simulink model "Tipo4_v4"  (R2018b)
settings: Solver=FixedStepDiscrete  StartTime=0.0  StopTime=50.3  MaxStep=50e-6  RelTol=1e-3
PreLoadFcn:
  | Ts=2e-6;
InitFcn:
  | %xInitial = init_power_wind_dfig_det;
  | Ts=2e-6;
undefined symbols (not defined in the file): D1, Delta, DiscIntNeverNeededParam, find_system
libraries: powerlib x144, simulink x110, powerlib_meascontrol x83, simulink_extras x6, powerlib_extras x4
(part 3 of 6)

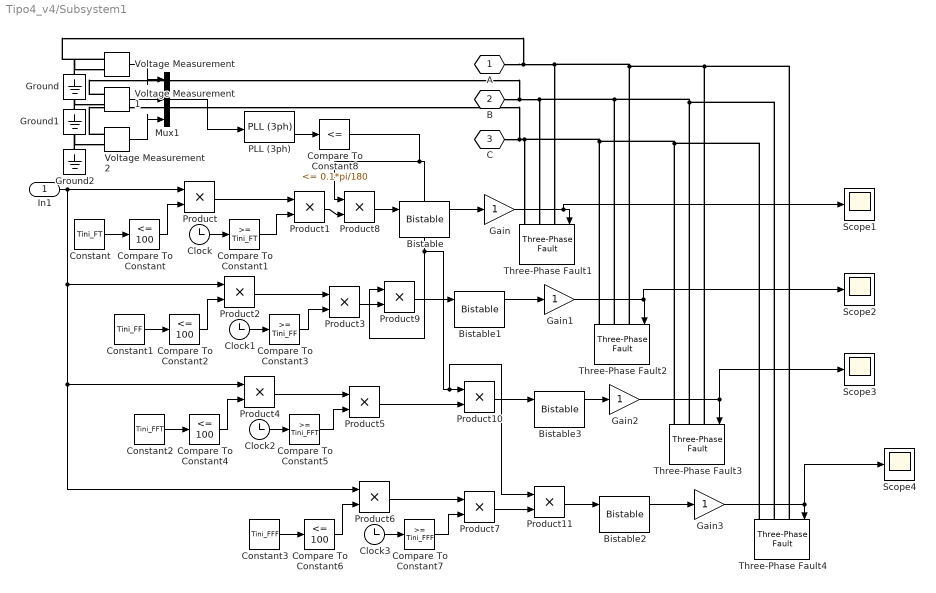
== system Tipo4_v4/Subsystem1 ==
  In1 : Inport
  Bistable{,1..3} (4 alike) : powerlib_meascontrol/Logic/Bistable  Qpriority=Set  ic=0  Ts=Ts
      settings: SourceProductName=Simscape Power Systems  SourceProductBaseCode=PS
  Clock{,1..3} (4 alike) : Clock
  Compare To Constant{,2,4,6} (4 alike) : simulink/Logic and Bit Operations/Compare To Constant  relop=<=  const=100  OutDataTypeStr=uint8
  Compare To Constant1 : simulink/Logic and Bit Operations/Compare To Constant  relop=>=  const=Tini_FT  OutDataTypeStr=uint8
  Compare To Constant3 : simulink/Logic and Bit Operations/Compare To Constant  relop=>=  const=Tini_FF  OutDataTypeStr=uint8
  Compare To Constant5 : simulink/Logic and Bit Operations/Compare To Constant  relop=>=  const=Tini_FFT  OutDataTypeStr=uint8
  Compare To Constant7 : simulink/Logic and Bit Operations/Compare To Constant  relop=>=  const=Tini_FFF  OutDataTypeStr=uint8
  Compare To Constant8 : simulink/Logic and Bit Operations/Compare To Constant  relop=<=  const=0.1*pi/180  OutDataTypeStr=uint8
  Constant : Constant  Value=Tini_FT
  Constant1 : Constant  Value=Tini_FF
  Constant2 : Constant  Value=Tini_FFT
  Constant3 : Constant  Value=Tini_FFF
  Gain{,1..3} (4 alike) : Gain  OutDataTypeStr=double
  Ground : powerlib/Elements/Ground  LConnTagsString=a
  Ground1 : powerlib/Elements/Ground  LConnTagsString=a
  Ground2 : powerlib/Elements/Ground  LConnTagsString=a
  Mux1 : Mux  Inputs=3
  PLL (3ph) : powerlib_meascontrol/PLL/PLL (3ph)  Fmin=60  Par_Init=[0, 60]  ParK=[180, 3200, 1]  TcD=1e-4  MaxRateChangeFreq=12  FilterCutOffFreq=25  Ts=Ts  AGC=on
  Product{,2..7} (7 alike) : Product
  Product{1,8..11} (5 alike) : Product  RndMeth=Ceiling
  Scope{1..4} (4 alike) : Scope
  Three-Phase Fault1 : powerlib/Elements/Three-Phase Fault  InitialStates=0  FaultA=on  FaultB=off  FaultC=off  GroundFault=on  SwitchTimes=[900 1000]  External=on  SwitchStatus=NaN  FaultResistance=R_falta  GroundResistance=R_falta  SnubberResistance=1e6  SnubberCapacitance=inf  Measurements=None
  Three-Phase Fault2 : powerlib/Elements/Three-Phase Fault  InitialStates=0  FaultA=on  FaultB=on  FaultC=off  GroundFault=off  SwitchTimes=[900 1000]  External=on  SwitchStatus=NaN  FaultResistance=R_falta  GroundResistance=1e-12  SnubberResistance=1e6  SnubberCapacitance=inf  Measurements=None
  Three-Phase Fault3 : powerlib/Elements/Three-Phase Fault  InitialStates=0  FaultA=on  FaultB=on  FaultC=off  GroundFault=on  SwitchTimes=[900 1000]  External=on  SwitchStatus=NaN  FaultResistance=R_falta  GroundResistance=R_falta  SnubberResistance=1e6  SnubberCapacitance=inf  Measurements=None
  Three-Phase Fault4 : powerlib/Elements/Three-Phase Fault  InitialStates=0  FaultA=on  FaultB=on  FaultC=on  GroundFault=on  SwitchTimes=[900 1000]  External=on  SwitchStatus=NaN  FaultResistance=R_falta  GroundResistance=R_falta  SnubberResistance=1e6  SnubberCapacitance=inf  Measurements=None
  Voltage Measurement : powerlib/Measurements/Voltage Measurement  PhasorSimulation=off  OutputType=Complex  PSBequivalent=0
  Voltage Measurement1 : powerlib/Measurements/Voltage Measurement  PhasorSimulation=off  OutputType=Complex  PSBequivalent=0
  Voltage Measurement2 : powerlib/Measurements/Voltage Measurement  PhasorSimulation=off  OutputType=Complex  PSBequivalent=0
  A : PMIOPort  Tag=PMCPort  Side=Right
  B : PMIOPort  Tag=PMCPort  Port=2  Side=Right
  C : PMIOPort  Tag=PMCPort  Port=3  Side=Right
  wires:
  Clock/1 -> Compare To Constant1/1
  Product2/1 -> Product3/1
  Constant1/1 -> Compare To Constant2/1
  Product/1 -> Product1/1
  Compare To Constant2/1 -> Product2/2
  Constant2/1 -> Compare To Constant4/1
  Clock2/1 -> Compare To Constant5/1
  Compare To Constant4/1 -> Product4/2
  Clock1/1 -> Compare To Constant3/1
  Compare To Constant5/1 -> Product5/2
  In1/1 -> Product/1, Product2/1, Product4/1, Product6/1
  Clock3/1 -> Compare To Constant7/1
  Constant3/1 -> Compare To Constant6/1
  Compare To Constant6/1 -> Product6/2
  Product6/1 -> Product7/1
  Compare To Constant7/1 -> Product7/2
  Compare To Constant3/1 -> Product3/2
  Constant/1 -> Compare To Constant/1
  Compare To Constant/1 -> Product/2
  Compare To Constant1/1 -> Product1/2
  Product4/1 -> Product5/1
  Product1/1 -> Product8/2
  Product8/1 -> Bistable/1
  Product3/1 -> Product9/2
  Product5/1 -> Product10/2
  Product7/1 -> Product11/2
  Compare To Constant8/1 -> Product11/1, Product10/1, Product9/1, Product8/1
  PLL (3ph)/2 -> Compare To Constant8/1
  Voltage Measurement1/1 -> Mux1/2
  Voltage Measurement/1 -> Mux1/1
  Voltage Measurement2/1 -> Mux1/3
  Mux1/1 -> PLL (3ph)/1
  Gain/1 -> Scope1/1, Three-Phase Fault1/1
  Gain1/1 -> Scope2/1, Three-Phase Fault2/1
  Gain2/1 -> Three-Phase Fault3/1, Scope3/1
  Gain3/1 -> Scope4/1, Three-Phase Fault4/1
  Bistable/1 -> Gain/1
  Product9/1 -> Bistable1/1
  Bistable1/1 -> Gain1/1
  Bistable3/1 -> Gain2/1
  Product10/1 -> Bistable3/1
  Product11/1 -> Bistable2/1
  Bistable2/1 -> Gain3/1
  connections:
  Voltage Measurement1/LConn1 -- B/RConn1 -- Three-Phase Fault1/LConn2 -- Three-Phase Fault2/LConn2 -- Three-Phase Fault3/LConn2 -- Three-Phase Fault4/LConn2
  Voltage Measurement2/LConn1 -- C/RConn1 -- Three-Phase Fault4/LConn3 -- Three-Phase Fault3/LConn3 -- Three-Phase Fault2/LConn3 -- Three-Phase Fault1/LConn3
  A/RConn1 -- Voltage Measurement/LConn1 -- Three-Phase Fault1/LConn1 -- Three-Phase Fault2/LConn1 -- Three-Phase Fault3/LConn1 -- Three-Phase Fault4/LConn1
  Ground/LConn1 -- Voltage Measurement/LConn2
  Ground1/LConn1 -- Voltage Measurement1/LConn2
  Ground2/LConn1 -- Voltage Measurement2/LConn2

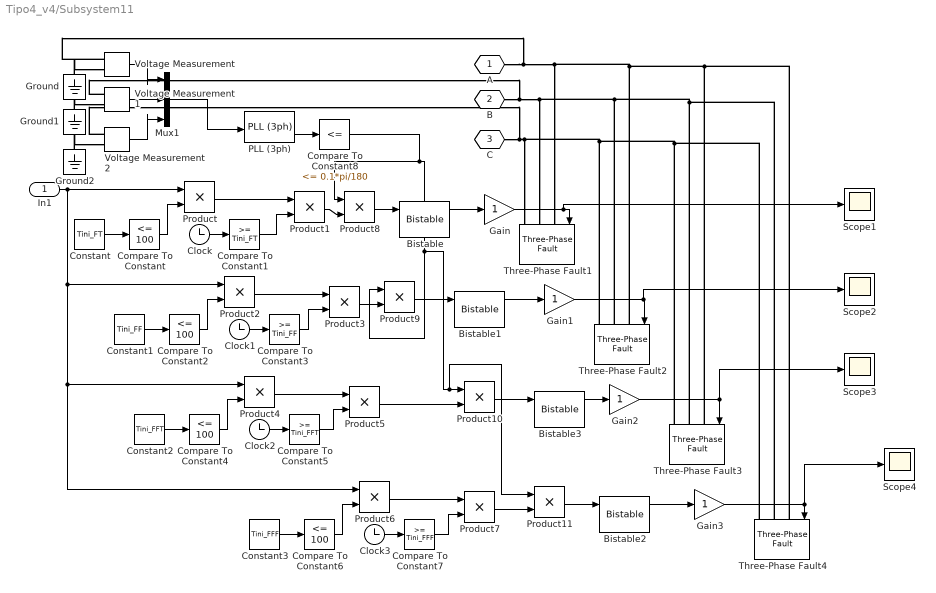
== system Tipo4_v4/Subsystem11 ==
  In1 : Inport
  Bistable{,1..3} (4 alike) : powerlib_meascontrol/Logic/Bistable  Qpriority=Set  ic=0  Ts=Ts
      settings: SourceProductName=Simscape Power Systems  SourceProductBaseCode=PS
  Clock{,1..3} (4 alike) : Clock
  Compare To Constant{,2,4,6} (4 alike) : simulink/Logic and Bit Operations/Compare To Constant  relop=<=  const=100  OutDataTypeStr=uint8
  Compare To Constant1 : simulink/Logic and Bit Operations/Compare To Constant  relop=>=  const=Tini_FT  OutDataTypeStr=uint8
  Compare To Constant3 : simulink/Logic and Bit Operations/Compare To Constant  relop=>=  const=Tini_FF  OutDataTypeStr=uint8
  Compare To Constant5 : simulink/Logic and Bit Operations/Compare To Constant  relop=>=  const=Tini_FFT  OutDataTypeStr=uint8
  Compare To Constant7 : simulink/Logic and Bit Operations/Compare To Constant  relop=>=  const=Tini_FFF  OutDataTypeStr=uint8
  Compare To Constant8 : simulink/Logic and Bit Operations/Compare To Constant  relop=<=  const=0.1*pi/180  OutDataTypeStr=uint8
  Constant : Constant  Value=Tini_FT
  Constant1 : Constant  Value=Tini_FF
  Constant2 : Constant  Value=Tini_FFT
  Constant3 : Constant  Value=Tini_FFF
  Gain{,1..3} (4 alike) : Gain  OutDataTypeStr=double
  Ground : powerlib/Elements/Ground  LConnTagsString=a
  Ground1 : powerlib/Elements/Ground  LConnTagsString=a
  Ground2 : powerlib/Elements/Ground  LConnTagsString=a
  Mux1 : Mux  Inputs=3
  PLL (3ph) : powerlib_meascontrol/PLL/PLL (3ph)  Fmin=60  Par_Init=[0, 60]  ParK=[180, 3200, 1]  TcD=1e-4  MaxRateChangeFreq=12  FilterCutOffFreq=25  Ts=Ts  AGC=on
  Product{,2..7} (7 alike) : Product
  Product{1,8..11} (5 alike) : Product  RndMeth=Ceiling
  Scope{1..4} (4 alike) : Scope
  Three-Phase Fault1 : powerlib/Elements/Three-Phase Fault  InitialStates=0  FaultA=on  FaultB=off  FaultC=off  GroundFault=on  SwitchTimes=[900 1000]  External=on  SwitchStatus=NaN  FaultResistance=R_falta  GroundResistance=R_falta  SnubberResistance=1e6  SnubberCapacitance=inf  Measurements=None
  Three-Phase Fault2 : powerlib/Elements/Three-Phase Fault  InitialStates=0  FaultA=on  FaultB=on  FaultC=off  GroundFault=off  SwitchTimes=[900 1000]  External=on  SwitchStatus=NaN  FaultResistance=R_falta  GroundResistance=1e-12  SnubberResistance=1e6  SnubberCapacitance=inf  Measurements=None
  Three-Phase Fault3 : powerlib/Elements/Three-Phase Fault  InitialStates=0  FaultA=on  FaultB=on  FaultC=off  GroundFault=on  SwitchTimes=[900 1000]  External=on  SwitchStatus=NaN  FaultResistance=R_falta  GroundResistance=R_falta  SnubberResistance=1e6  SnubberCapacitance=inf  Measurements=None
  Three-Phase Fault4 : powerlib/Elements/Three-Phase Fault  InitialStates=0  FaultA=on  FaultB=on  FaultC=on  GroundFault=on  SwitchTimes=[900 1000]  External=on  SwitchStatus=NaN  FaultResistance=R_falta  GroundResistance=R_falta  SnubberResistance=1e6  SnubberCapacitance=inf  Measurements=None
  Voltage Measurement : powerlib/Measurements/Voltage Measurement  PhasorSimulation=off  OutputType=Complex  PSBequivalent=0
  Voltage Measurement1 : powerlib/Measurements/Voltage Measurement  PhasorSimulation=off  OutputType=Complex  PSBequivalent=0
  Voltage Measurement2 : powerlib/Measurements/Voltage Measurement  PhasorSimulation=off  OutputType=Complex  PSBequivalent=0
  A : PMIOPort  Tag=PMCPort  Side=Right
  B : PMIOPort  Tag=PMCPort  Port=2  Side=Right
  C : PMIOPort  Tag=PMCPort  Port=3  Side=Right
  wires:
  Clock/1 -> Compare To Constant1/1
  Product2/1 -> Product3/1
  Constant1/1 -> Compare To Constant2/1
  Product/1 -> Product1/1
  Compare To Constant2/1 -> Product2/2
  Constant2/1 -> Compare To Constant4/1
  Clock2/1 -> Compare To Constant5/1
  Compare To Constant4/1 -> Product4/2
  Clock1/1 -> Compare To Constant3/1
  Compare To Constant5/1 -> Product5/2
  In1/1 -> Product/1, Product2/1, Product4/1, Product6/1
  Clock3/1 -> Compare To Constant7/1
  Constant3/1 -> Compare To Constant6/1
  Compare To Constant6/1 -> Product6/2
  Product6/1 -> Product7/1
  Compare To Constant7/1 -> Product7/2
  Compare To Constant3/1 -> Product3/2
  Constant/1 -> Compare To Constant/1
  Compare To Constant/1 -> Product/2
  Compare To Constant1/1 -> Product1/2
  Product4/1 -> Product5/1
  Product1/1 -> Product8/2
  Product8/1 -> Bistable/1
  Product3/1 -> Product9/2
  Product5/1 -> Product10/2
  Product7/1 -> Product11/2
  Compare To Constant8/1 -> Product11/1, Product10/1, Product9/1, Product8/1
  PLL (3ph)/2 -> Compare To Constant8/1
  Voltage Measurement1/1 -> Mux1/2
  Voltage Measurement/1 -> Mux1/1
  Voltage Measurement2/1 -> Mux1/3
  Mux1/1 -> PLL (3ph)/1
  Gain/1 -> Scope1/1, Three-Phase Fault1/1
  Gain1/1 -> Scope2/1, Three-Phase Fault2/1
  Gain2/1 -> Three-Phase Fault3/1, Scope3/1
  Gain3/1 -> Scope4/1, Three-Phase Fault4/1
  Bistable/1 -> Gain/1
  Product9/1 -> Bistable1/1
  Bistable1/1 -> Gain1/1
  Bistable3/1 -> Gain2/1
  Product10/1 -> Bistable3/1
  Product11/1 -> Bistable2/1
  Bistable2/1 -> Gain3/1
  connections:
  Voltage Measurement1/LConn1 -- B/RConn1 -- Three-Phase Fault1/LConn2 -- Three-Phase Fault2/LConn2 -- Three-Phase Fault3/LConn2 -- Three-Phase Fault4/LConn2
  Voltage Measurement2/LConn1 -- C/RConn1 -- Three-Phase Fault4/LConn3 -- Three-Phase Fault3/LConn3 -- Three-Phase Fault2/LConn3 -- Three-Phase Fault1/LConn3
  A/RConn1 -- Voltage Measurement/LConn1 -- Three-Phase Fault1/LConn1 -- Three-Phase Fault2/LConn1 -- Three-Phase Fault3/LConn1 -- Three-Phase Fault4/LConn1
  Ground/LConn1 -- Voltage Measurement/LConn2
  Ground1/LConn1 -- Voltage Measurement1/LConn2
  Ground2/LConn1 -- Voltage Measurement2/LConn2

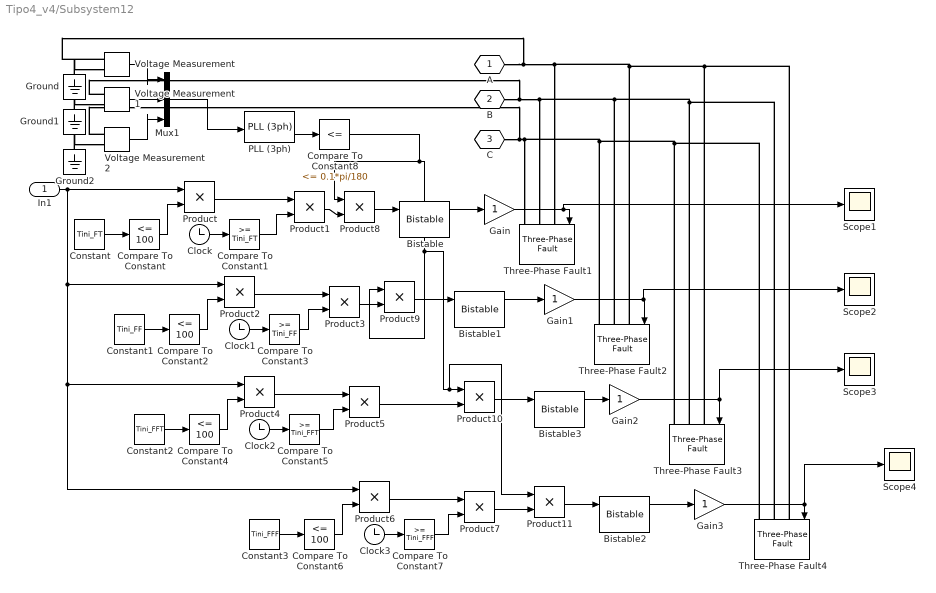
== system Tipo4_v4/Subsystem12 ==
  In1 : Inport
  Bistable{,1..3} (4 alike) : powerlib_meascontrol/Logic/Bistable  Qpriority=Set  ic=0  Ts=Ts
      settings: SourceProductName=Simscape Power Systems  SourceProductBaseCode=PS
  Clock{,1..3} (4 alike) : Clock
  Compare To Constant{,2,4,6} (4 alike) : simulink/Logic and Bit Operations/Compare To Constant  relop=<=  const=100  OutDataTypeStr=uint8
  Compare To Constant1 : simulink/Logic and Bit Operations/Compare To Constant  relop=>=  const=Tini_FT  OutDataTypeStr=uint8
  Compare To Constant3 : simulink/Logic and Bit Operations/Compare To Constant  relop=>=  const=Tini_FF  OutDataTypeStr=uint8
  Compare To Constant5 : simulink/Logic and Bit Operations/Compare To Constant  relop=>=  const=Tini_FFT  OutDataTypeStr=uint8
  Compare To Constant7 : simulink/Logic and Bit Operations/Compare To Constant  relop=>=  const=Tini_FFF  OutDataTypeStr=uint8
  Compare To Constant8 : simulink/Logic and Bit Operations/Compare To Constant  relop=<=  const=0.1*pi/180  OutDataTypeStr=uint8
  Constant : Constant  Value=Tini_FT
  Constant1 : Constant  Value=Tini_FF
  Constant2 : Constant  Value=Tini_FFT
  Constant3 : Constant  Value=Tini_FFF
  Gain{,1..3} (4 alike) : Gain  OutDataTypeStr=double
  Ground : powerlib/Elements/Ground  LConnTagsString=a
  Ground1 : powerlib/Elements/Ground  LConnTagsString=a
  Ground2 : powerlib/Elements/Ground  LConnTagsString=a
  Mux1 : Mux  Inputs=3
  PLL (3ph) : powerlib_meascontrol/PLL/PLL (3ph)  Fmin=60  Par_Init=[0, 60]  ParK=[180, 3200, 1]  TcD=1e-4  MaxRateChangeFreq=12  FilterCutOffFreq=25  Ts=Ts  AGC=on
  Product{,2..7} (7 alike) : Product
  Product{1,8..11} (5 alike) : Product  RndMeth=Ceiling
  Scope{1..4} (4 alike) : Scope
  Three-Phase Fault1 : powerlib/Elements/Three-Phase Fault  InitialStates=0  FaultA=on  FaultB=off  FaultC=off  GroundFault=on  SwitchTimes=[900 1000]  External=on  SwitchStatus=NaN  FaultResistance=R_falta  GroundResistance=R_falta  SnubberResistance=1e6  SnubberCapacitance=inf  Measurements=None
  Three-Phase Fault2 : powerlib/Elements/Three-Phase Fault  InitialStates=0  FaultA=on  FaultB=on  FaultC=off  GroundFault=off  SwitchTimes=[900 1000]  External=on  SwitchStatus=NaN  FaultResistance=R_falta  GroundResistance=1e-12  SnubberResistance=1e6  SnubberCapacitance=inf  Measurements=None
  Three-Phase Fault3 : powerlib/Elements/Three-Phase Fault  InitialStates=0  FaultA=on  FaultB=on  FaultC=off  GroundFault=on  SwitchTimes=[900 1000]  External=on  SwitchStatus=NaN  FaultResistance=R_falta  GroundResistance=R_falta  SnubberResistance=1e6  SnubberCapacitance=inf  Measurements=None
  Three-Phase Fault4 : powerlib/Elements/Three-Phase Fault  InitialStates=0  FaultA=on  FaultB=on  FaultC=on  GroundFault=on  SwitchTimes=[900 1000]  External=on  SwitchStatus=NaN  FaultResistance=R_falta  GroundResistance=R_falta  SnubberResistance=1e6  SnubberCapacitance=inf  Measurements=None
  Voltage Measurement : powerlib/Measurements/Voltage Measurement  PhasorSimulation=off  OutputType=Complex  PSBequivalent=0
  Voltage Measurement1 : powerlib/Measurements/Voltage Measurement  PhasorSimulation=off  OutputType=Complex  PSBequivalent=0
  Voltage Measurement2 : powerlib/Measurements/Voltage Measurement  PhasorSimulation=off  OutputType=Complex  PSBequivalent=0
  A : PMIOPort  Tag=PMCPort  Side=Right
  B : PMIOPort  Tag=PMCPort  Port=2  Side=Right
  C : PMIOPort  Tag=PMCPort  Port=3  Side=Right
  wires:
  Clock/1 -> Compare To Constant1/1
  Product2/1 -> Product3/1
  Constant1/1 -> Compare To Constant2/1
  Product/1 -> Product1/1
  Compare To Constant2/1 -> Product2/2
  Constant2/1 -> Compare To Constant4/1
  Clock2/1 -> Compare To Constant5/1
  Compare To Constant4/1 -> Product4/2
  Clock1/1 -> Compare To Constant3/1
  Compare To Constant5/1 -> Product5/2
  In1/1 -> Product/1, Product2/1, Product4/1, Product6/1
  Clock3/1 -> Compare To Constant7/1
  Constant3/1 -> Compare To Constant6/1
  Compare To Constant6/1 -> Product6/2
  Product6/1 -> Product7/1
  Compare To Constant7/1 -> Product7/2
  Compare To Constant3/1 -> Product3/2
  Constant/1 -> Compare To Constant/1
  Compare To Constant/1 -> Product/2
  Compare To Constant1/1 -> Product1/2
  Product4/1 -> Product5/1
  Product1/1 -> Product8/2
  Product8/1 -> Bistable/1
  Product3/1 -> Product9/2
  Product5/1 -> Product10/2
  Product7/1 -> Product11/2
  Compare To Constant8/1 -> Product11/1, Product10/1, Product9/1, Product8/1
  PLL (3ph)/2 -> Compare To Constant8/1
  Voltage Measurement1/1 -> Mux1/2
  Voltage Measurement/1 -> Mux1/1
  Voltage Measurement2/1 -> Mux1/3
  Mux1/1 -> PLL (3ph)/1
  Gain/1 -> Scope1/1, Three-Phase Fault1/1
  Gain1/1 -> Scope2/1, Three-Phase Fault2/1
  Gain2/1 -> Three-Phase Fault3/1, Scope3/1
  Gain3/1 -> Scope4/1, Three-Phase Fault4/1
  Bistable/1 -> Gain/1
  Product9/1 -> Bistable1/1
  Bistable1/1 -> Gain1/1
  Bistable3/1 -> Gain2/1
  Product10/1 -> Bistable3/1
  Product11/1 -> Bistable2/1
  Bistable2/1 -> Gain3/1
  connections:
  Voltage Measurement1/LConn1 -- B/RConn1 -- Three-Phase Fault1/LConn2 -- Three-Phase Fault2/LConn2 -- Three-Phase Fault3/LConn2 -- Three-Phase Fault4/LConn2
  Voltage Measurement2/LConn1 -- C/RConn1 -- Three-Phase Fault4/LConn3 -- Three-Phase Fault3/LConn3 -- Three-Phase Fault2/LConn3 -- Three-Phase Fault1/LConn3
  A/RConn1 -- Voltage Measurement/LConn1 -- Three-Phase Fault1/LConn1 -- Three-Phase Fault2/LConn1 -- Three-Phase Fault3/LConn1 -- Three-Phase Fault4/LConn1
  Ground/LConn1 -- Voltage Measurement/LConn2
  Ground1/LConn1 -- Voltage Measurement1/LConn2
  Ground2/LConn1 -- Voltage Measurement2/LConn2

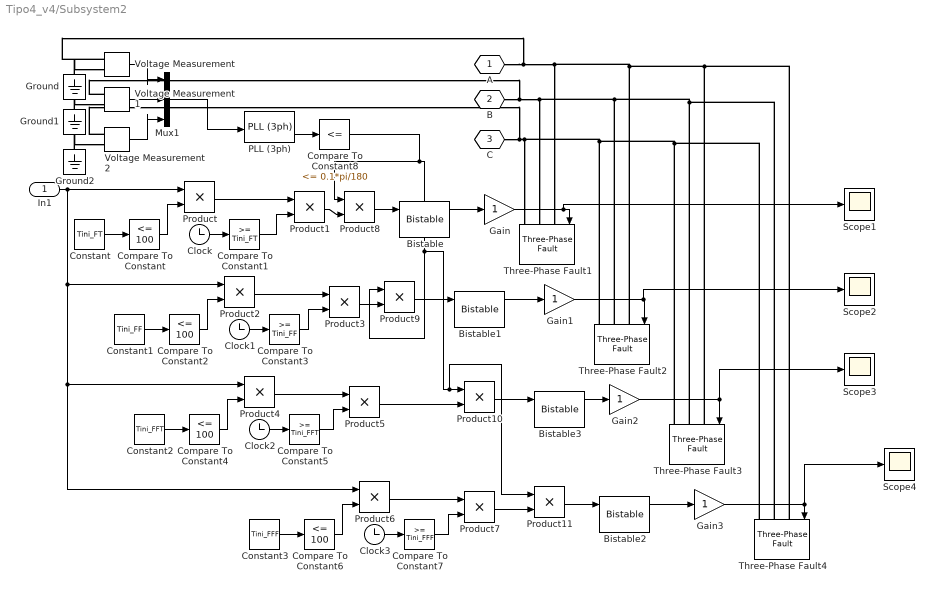
== system Tipo4_v4/Subsystem2 ==
  In1 : Inport
  Bistable{,1..3} (4 alike) : powerlib_meascontrol/Logic/Bistable  Qpriority=Set  ic=0  Ts=Ts
      settings: SourceProductName=Simscape Power Systems  SourceProductBaseCode=PS
  Clock{,1..3} (4 alike) : Clock
  Compare To Constant{,2,4,6} (4 alike) : simulink/Logic and Bit Operations/Compare To Constant  relop=<=  const=100  OutDataTypeStr=uint8
  Compare To Constant1 : simulink/Logic and Bit Operations/Compare To Constant  relop=>=  const=Tini_FT  OutDataTypeStr=uint8
  Compare To Constant3 : simulink/Logic and Bit Operations/Compare To Constant  relop=>=  const=Tini_FF  OutDataTypeStr=uint8
  Compare To Constant5 : simulink/Logic and Bit Operations/Compare To Constant  relop=>=  const=Tini_FFT  OutDataTypeStr=uint8
  Compare To Constant7 : simulink/Logic and Bit Operations/Compare To Constant  relop=>=  const=Tini_FFF  OutDataTypeStr=uint8
  Compare To Constant8 : simulink/Logic and Bit Operations/Compare To Constant  relop=<=  const=0.1*pi/180  OutDataTypeStr=uint8
  Constant : Constant  Value=Tini_FT
  Constant1 : Constant  Value=Tini_FF
  Constant2 : Constant  Value=Tini_FFT
  Constant3 : Constant  Value=Tini_FFF
  Gain{,1..3} (4 alike) : Gain  OutDataTypeStr=double
  Ground : powerlib/Elements/Ground  LConnTagsString=a
  Ground1 : powerlib/Elements/Ground  LConnTagsString=a
  Ground2 : powerlib/Elements/Ground  LConnTagsString=a
  Mux1 : Mux  Inputs=3
  PLL (3ph) : powerlib_meascontrol/PLL/PLL (3ph)  Fmin=60  Par_Init=[0, 60]  ParK=[180, 3200, 1]  TcD=1e-4  MaxRateChangeFreq=12  FilterCutOffFreq=25  Ts=Ts  AGC=on
  Product{,2..7} (7 alike) : Product
  Product{1,8..11} (5 alike) : Product  RndMeth=Ceiling
  Scope{1..4} (4 alike) : Scope
  Three-Phase Fault1 : powerlib/Elements/Three-Phase Fault  InitialStates=0  FaultA=on  FaultB=off  FaultC=off  GroundFault=on  SwitchTimes=[900 1000]  External=on  SwitchStatus=NaN  FaultResistance=R_falta  GroundResistance=R_falta  SnubberResistance=1e6  SnubberCapacitance=inf  Measurements=None
  Three-Phase Fault2 : powerlib/Elements/Three-Phase Fault  InitialStates=0  FaultA=on  FaultB=on  FaultC=off  GroundFault=off  SwitchTimes=[900 1000]  External=on  SwitchStatus=NaN  FaultResistance=R_falta  GroundResistance=1e-12  SnubberResistance=1e6  SnubberCapacitance=inf  Measurements=None
  Three-Phase Fault3 : powerlib/Elements/Three-Phase Fault  InitialStates=0  FaultA=on  FaultB=on  FaultC=off  GroundFault=on  SwitchTimes=[900 1000]  External=on  SwitchStatus=NaN  FaultResistance=R_falta  GroundResistance=R_falta  SnubberResistance=1e6  SnubberCapacitance=inf  Measurements=None
  Three-Phase Fault4 : powerlib/Elements/Three-Phase Fault  InitialStates=0  FaultA=on  FaultB=on  FaultC=on  GroundFault=on  SwitchTimes=[900 1000]  External=on  SwitchStatus=NaN  FaultResistance=R_falta  GroundResistance=R_falta  SnubberResistance=1e6  SnubberCapacitance=inf  Measurements=None
  Voltage Measurement : powerlib/Measurements/Voltage Measurement  PhasorSimulation=off  OutputType=Complex  PSBequivalent=0
  Voltage Measurement1 : powerlib/Measurements/Voltage Measurement  PhasorSimulation=off  OutputType=Complex  PSBequivalent=0
  Voltage Measurement2 : powerlib/Measurements/Voltage Measurement  PhasorSimulation=off  OutputType=Complex  PSBequivalent=0
  A : PMIOPort  Tag=PMCPort  Side=Right
  B : PMIOPort  Tag=PMCPort  Port=2  Side=Right
  C : PMIOPort  Tag=PMCPort  Port=3  Side=Right
  wires:
  Clock/1 -> Compare To Constant1/1
  Product2/1 -> Product3/1
  Constant1/1 -> Compare To Constant2/1
  Product/1 -> Product1/1
  Compare To Constant2/1 -> Product2/2
  Constant2/1 -> Compare To Constant4/1
  Clock2/1 -> Compare To Constant5/1
  Compare To Constant4/1 -> Product4/2
  Clock1/1 -> Compare To Constant3/1
  Compare To Constant5/1 -> Product5/2
  In1/1 -> Product/1, Product2/1, Product4/1, Product6/1
  Clock3/1 -> Compare To Constant7/1
  Constant3/1 -> Compare To Constant6/1
  Compare To Constant6/1 -> Product6/2
  Product6/1 -> Product7/1
  Compare To Constant7/1 -> Product7/2
  Compare To Constant3/1 -> Product3/2
  Constant/1 -> Compare To Constant/1
  Compare To Constant/1 -> Product/2
  Compare To Constant1/1 -> Product1/2
  Product4/1 -> Product5/1
  Product1/1 -> Product8/2
  Product8/1 -> Bistable/1
  Product3/1 -> Product9/2
  Product5/1 -> Product10/2
  Product7/1 -> Product11/2
  Compare To Constant8/1 -> Product11/1, Product10/1, Product9/1, Product8/1
  PLL (3ph)/2 -> Compare To Constant8/1
  Voltage Measurement1/1 -> Mux1/2
  Voltage Measurement/1 -> Mux1/1
  Voltage Measurement2/1 -> Mux1/3
  Mux1/1 -> PLL (3ph)/1
  Gain/1 -> Scope1/1, Three-Phase Fault1/1
  Gain1/1 -> Scope2/1, Three-Phase Fault2/1
  Gain2/1 -> Three-Phase Fault3/1, Scope3/1
  Gain3/1 -> Scope4/1, Three-Phase Fault4/1
  Bistable/1 -> Gain/1
  Product9/1 -> Bistable1/1
  Bistable1/1 -> Gain1/1
  Bistable3/1 -> Gain2/1
  Product10/1 -> Bistable3/1
  Product11/1 -> Bistable2/1
  Bistable2/1 -> Gain3/1
  connections:
  Voltage Measurement1/LConn1 -- B/RConn1 -- Three-Phase Fault1/LConn2 -- Three-Phase Fault2/LConn2 -- Three-Phase Fault3/LConn2 -- Three-Phase Fault4/LConn2
  Voltage Measurement2/LConn1 -- C/RConn1 -- Three-Phase Fault4/LConn3 -- Three-Phase Fault3/LConn3 -- Three-Phase Fault2/LConn3 -- Three-Phase Fault1/LConn3
  A/RConn1 -- Voltage Measurement/LConn1 -- Three-Phase Fault1/LConn1 -- Three-Phase Fault2/LConn1 -- Three-Phase Fault3/LConn1 -- Three-Phase Fault4/LConn1
  Ground/LConn1 -- Voltage Measurement/LConn2
  Ground1/LConn1 -- Voltage Measurement1/LConn2
  Ground2/LConn1 -- Voltage Measurement2/LConn2

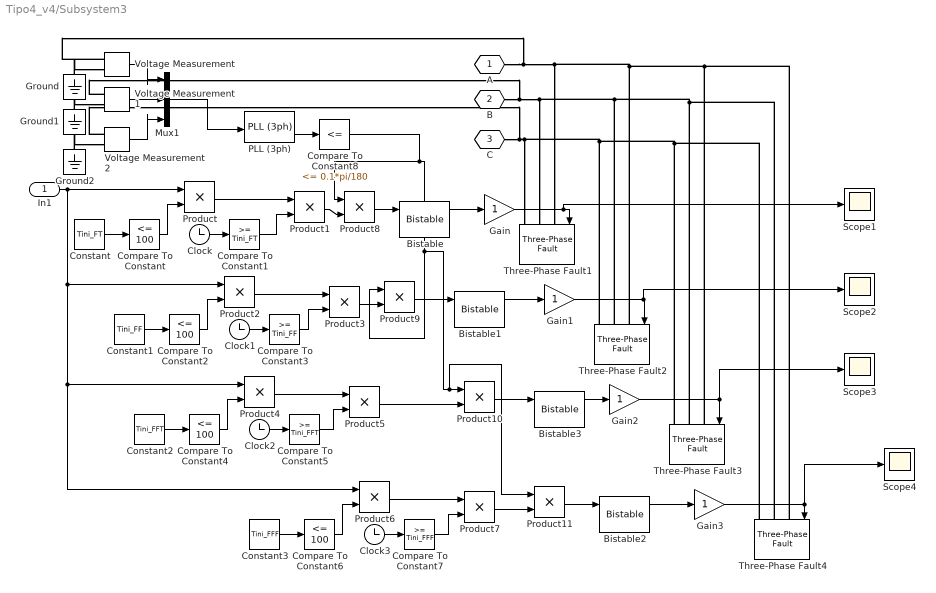
== system Tipo4_v4/Subsystem3 ==
  In1 : Inport
  Bistable{,1..3} (4 alike) : powerlib_meascontrol/Logic/Bistable  Qpriority=Set  ic=0  Ts=Ts
      settings: SourceProductName=Simscape Power Systems  SourceProductBaseCode=PS
  Clock{,1..3} (4 alike) : Clock
  Compare To Constant{,2,4,6} (4 alike) : simulink/Logic and Bit Operations/Compare To Constant  relop=<=  const=100  OutDataTypeStr=uint8
  Compare To Constant1 : simulink/Logic and Bit Operations/Compare To Constant  relop=>=  const=Tini_FT  OutDataTypeStr=uint8
  Compare To Constant3 : simulink/Logic and Bit Operations/Compare To Constant  relop=>=  const=Tini_FF  OutDataTypeStr=uint8
  Compare To Constant5 : simulink/Logic and Bit Operations/Compare To Constant  relop=>=  const=Tini_FFT  OutDataTypeStr=uint8
  Compare To Constant7 : simulink/Logic and Bit Operations/Compare To Constant  relop=>=  const=Tini_FFF  OutDataTypeStr=uint8
  Compare To Constant8 : simulink/Logic and Bit Operations/Compare To Constant  relop=<=  const=0.1*pi/180  OutDataTypeStr=uint8
  Constant : Constant  Value=Tini_FT
  Constant1 : Constant  Value=Tini_FF
  Constant2 : Constant  Value=Tini_FFT
  Constant3 : Constant  Value=Tini_FFF
  Gain{,1..3} (4 alike) : Gain  OutDataTypeStr=double
  Ground : powerlib/Elements/Ground  LConnTagsString=a
  Ground1 : powerlib/Elements/Ground  LConnTagsString=a
  Ground2 : powerlib/Elements/Ground  LConnTagsString=a
  Mux1 : Mux  Inputs=3
  PLL (3ph) : powerlib_meascontrol/PLL/PLL (3ph)  Fmin=60  Par_Init=[0, 60]  ParK=[180, 3200, 1]  TcD=1e-4  MaxRateChangeFreq=12  FilterCutOffFreq=25  Ts=Ts  AGC=on
  Product{,2..7} (7 alike) : Product
  Product{1,8..11} (5 alike) : Product  RndMeth=Ceiling
  Scope{1..4} (4 alike) : Scope
  Three-Phase Fault1 : powerlib/Elements/Three-Phase Fault  InitialStates=0  FaultA=on  FaultB=off  FaultC=off  GroundFault=on  SwitchTimes=[900 1000]  External=on  SwitchStatus=NaN  FaultResistance=R_falta  GroundResistance=R_falta  SnubberResistance=1e6  SnubberCapacitance=inf  Measurements=None
  Three-Phase Fault2 : powerlib/Elements/Three-Phase Fault  InitialStates=0  FaultA=on  FaultB=on  FaultC=off  GroundFault=off  SwitchTimes=[900 1000]  External=on  SwitchStatus=NaN  FaultResistance=R_falta  GroundResistance=1e-12  SnubberResistance=1e6  SnubberCapacitance=inf  Measurements=None
  Three-Phase Fault3 : powerlib/Elements/Three-Phase Fault  InitialStates=0  FaultA=on  FaultB=on  FaultC=off  GroundFault=on  SwitchTimes=[900 1000]  External=on  SwitchStatus=NaN  FaultResistance=R_falta  GroundResistance=R_falta  SnubberResistance=1e6  SnubberCapacitance=inf  Measurements=None
  Three-Phase Fault4 : powerlib/Elements/Three-Phase Fault  InitialStates=0  FaultA=on  FaultB=on  FaultC=on  GroundFault=on  SwitchTimes=[900 1000]  External=on  SwitchStatus=NaN  FaultResistance=R_falta  GroundResistance=R_falta  SnubberResistance=1e6  SnubberCapacitance=inf  Measurements=None
  Voltage Measurement : powerlib/Measurements/Voltage Measurement  PhasorSimulation=off  OutputType=Complex  PSBequivalent=0
  Voltage Measurement1 : powerlib/Measurements/Voltage Measurement  PhasorSimulation=off  OutputType=Complex  PSBequivalent=0
  Voltage Measurement2 : powerlib/Measurements/Voltage Measurement  PhasorSimulation=off  OutputType=Complex  PSBequivalent=0
  A : PMIOPort  Tag=PMCPort  Side=Right
  B : PMIOPort  Tag=PMCPort  Port=2  Side=Right
  C : PMIOPort  Tag=PMCPort  Port=3  Side=Right
  wires:
  Clock/1 -> Compare To Constant1/1
  Product2/1 -> Product3/1
  Constant1/1 -> Compare To Constant2/1
  Product/1 -> Product1/1
  Compare To Constant2/1 -> Product2/2
  Constant2/1 -> Compare To Constant4/1
  Clock2/1 -> Compare To Constant5/1
  Compare To Constant4/1 -> Product4/2
  Clock1/1 -> Compare To Constant3/1
  Compare To Constant5/1 -> Product5/2
  In1/1 -> Product/1, Product2/1, Product4/1, Product6/1
  Clock3/1 -> Compare To Constant7/1
  Constant3/1 -> Compare To Constant6/1
  Compare To Constant6/1 -> Product6/2
  Product6/1 -> Product7/1
  Compare To Constant7/1 -> Product7/2
  Compare To Constant3/1 -> Product3/2
  Constant/1 -> Compare To Constant/1
  Compare To Constant/1 -> Product/2
  Compare To Constant1/1 -> Product1/2
  Product4/1 -> Product5/1
  Product1/1 -> Product8/2
  Product8/1 -> Bistable/1
  Product3/1 -> Product9/2
  Product5/1 -> Product10/2
  Product7/1 -> Product11/2
  Compare To Constant8/1 -> Product11/1, Product10/1, Product9/1, Product8/1
  PLL (3ph)/2 -> Compare To Constant8/1
  Voltage Measurement1/1 -> Mux1/2
  Voltage Measurement/1 -> Mux1/1
  Voltage Measurement2/1 -> Mux1/3
  Mux1/1 -> PLL (3ph)/1
  Gain/1 -> Scope1/1, Three-Phase Fault1/1
  Gain1/1 -> Scope2/1, Three-Phase Fault2/1
  Gain2/1 -> Three-Phase Fault3/1, Scope3/1
  Gain3/1 -> Scope4/1, Three-Phase Fault4/1
  Bistable/1 -> Gain/1
  Product9/1 -> Bistable1/1
  Bistable1/1 -> Gain1/1
  Bistable3/1 -> Gain2/1
  Product10/1 -> Bistable3/1
  Product11/1 -> Bistable2/1
  Bistable2/1 -> Gain3/1
  connections:
  Voltage Measurement1/LConn1 -- B/RConn1 -- Three-Phase Fault1/LConn2 -- Three-Phase Fault2/LConn2 -- Three-Phase Fault3/LConn2 -- Three-Phase Fault4/LConn2
  Voltage Measurement2/LConn1 -- C/RConn1 -- Three-Phase Fault4/LConn3 -- Three-Phase Fault3/LConn3 -- Three-Phase Fault2/LConn3 -- Three-Phase Fault1/LConn3
  A/RConn1 -- Voltage Measurement/LConn1 -- Three-Phase Fault1/LConn1 -- Three-Phase Fault2/LConn1 -- Three-Phase Fault3/LConn1 -- Three-Phase Fault4/LConn1
  Ground/LConn1 -- Voltage Measurement/LConn2
  Ground1/LConn1 -- Voltage Measurement1/LConn2
  Ground2/LConn1 -- Voltage Measurement2/LConn2

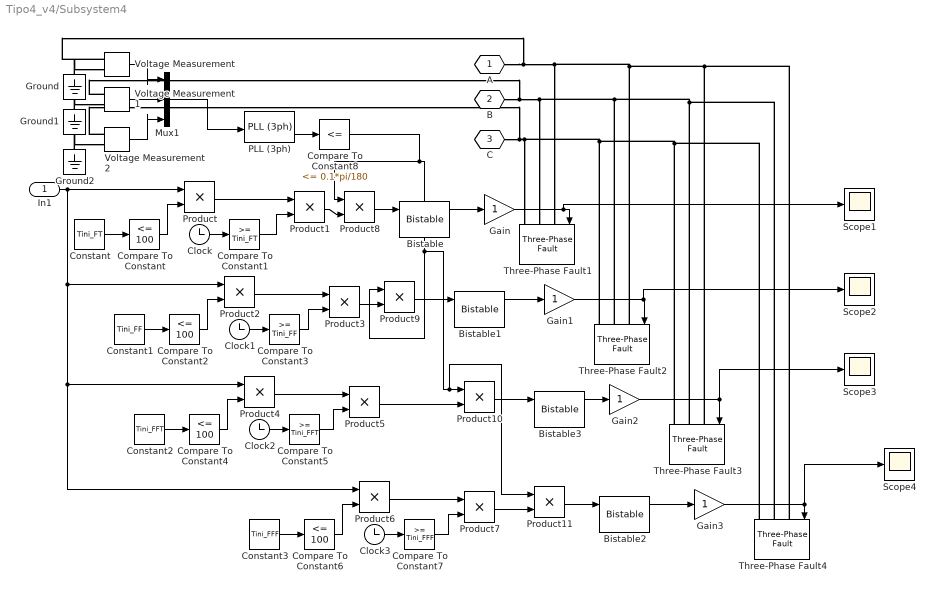
== system Tipo4_v4/Subsystem4 ==
  In1 : Inport
  Bistable{,1..3} (4 alike) : powerlib_meascontrol/Logic/Bistable  Qpriority=Set  ic=0  Ts=Ts
      settings: SourceProductName=Simscape Power Systems  SourceProductBaseCode=PS
  Clock{,1..3} (4 alike) : Clock
  Compare To Constant{,2,4,6} (4 alike) : simulink/Logic and Bit Operations/Compare To Constant  relop=<=  const=100  OutDataTypeStr=uint8
  Compare To Constant1 : simulink/Logic and Bit Operations/Compare To Constant  relop=>=  const=Tini_FT  OutDataTypeStr=uint8
  Compare To Constant3 : simulink/Logic and Bit Operations/Compare To Constant  relop=>=  const=Tini_FF  OutDataTypeStr=uint8
  Compare To Constant5 : simulink/Logic and Bit Operations/Compare To Constant  relop=>=  const=Tini_FFT  OutDataTypeStr=uint8
  Compare To Constant7 : simulink/Logic and Bit Operations/Compare To Constant  relop=>=  const=Tini_FFF  OutDataTypeStr=uint8
  Compare To Constant8 : simulink/Logic and Bit Operations/Compare To Constant  relop=<=  const=0.1*pi/180  OutDataTypeStr=uint8
  Constant : Constant  Value=Tini_FT
  Constant1 : Constant  Value=Tini_FF
  Constant2 : Constant  Value=Tini_FFT
  Constant3 : Constant  Value=Tini_FFF
  Gain{,1..3} (4 alike) : Gain  OutDataTypeStr=double
  Ground : powerlib/Elements/Ground  LConnTagsString=a
  Ground1 : powerlib/Elements/Ground  LConnTagsString=a
  Ground2 : powerlib/Elements/Ground  LConnTagsString=a
  Mux1 : Mux  Inputs=3
  PLL (3ph) : powerlib_meascontrol/PLL/PLL (3ph)  Fmin=60  Par_Init=[0, 60]  ParK=[180, 3200, 1]  TcD=1e-4  MaxRateChangeFreq=12  FilterCutOffFreq=25  Ts=Ts  AGC=on
  Product{,2..7} (7 alike) : Product
  Product{1,8..11} (5 alike) : Product  RndMeth=Ceiling
  Scope{1..4} (4 alike) : Scope
  Three-Phase Fault1 : powerlib/Elements/Three-Phase Fault  InitialStates=0  FaultA=on  FaultB=off  FaultC=off  GroundFault=on  SwitchTimes=[900 1000]  External=on  SwitchStatus=NaN  FaultResistance=R_falta  GroundResistance=R_falta  SnubberResistance=1e6  SnubberCapacitance=inf  Measurements=None
  Three-Phase Fault2 : powerlib/Elements/Three-Phase Fault  InitialStates=0  FaultA=on  FaultB=on  FaultC=off  GroundFault=off  SwitchTimes=[900 1000]  External=on  SwitchStatus=NaN  FaultResistance=R_falta  GroundResistance=1e-12  SnubberResistance=1e6  SnubberCapacitance=inf  Measurements=None
  Three-Phase Fault3 : powerlib/Elements/Three-Phase Fault  InitialStates=0  FaultA=on  FaultB=on  FaultC=off  GroundFault=on  SwitchTimes=[900 1000]  External=on  SwitchStatus=NaN  FaultResistance=R_falta  GroundResistance=R_falta  SnubberResistance=1e6  SnubberCapacitance=inf  Measurements=None
  Three-Phase Fault4 : powerlib/Elements/Three-Phase Fault  InitialStates=0  FaultA=on  FaultB=on  FaultC=on  GroundFault=on  SwitchTimes=[900 1000]  External=on  SwitchStatus=NaN  FaultResistance=R_falta  GroundResistance=R_falta  SnubberResistance=1e6  SnubberCapacitance=inf  Measurements=None
  Voltage Measurement : powerlib/Measurements/Voltage Measurement  PhasorSimulation=off  OutputType=Complex  PSBequivalent=0
  Voltage Measurement1 : powerlib/Measurements/Voltage Measurement  PhasorSimulation=off  OutputType=Complex  PSBequivalent=0
  Voltage Measurement2 : powerlib/Measurements/Voltage Measurement  PhasorSimulation=off  OutputType=Complex  PSBequivalent=0
  A : PMIOPort  Tag=PMCPort  Side=Right
  B : PMIOPort  Tag=PMCPort  Port=2  Side=Right
  C : PMIOPort  Tag=PMCPort  Port=3  Side=Right
  wires:
  Clock/1 -> Compare To Constant1/1
  Product2/1 -> Product3/1
  Constant1/1 -> Compare To Constant2/1
  Product/1 -> Product1/1
  Compare To Constant2/1 -> Product2/2
  Constant2/1 -> Compare To Constant4/1
  Clock2/1 -> Compare To Constant5/1
  Compare To Constant4/1 -> Product4/2
  Clock1/1 -> Compare To Constant3/1
  Compare To Constant5/1 -> Product5/2
  In1/1 -> Product/1, Product2/1, Product4/1, Product6/1
  Clock3/1 -> Compare To Constant7/1
  Constant3/1 -> Compare To Constant6/1
  Compare To Constant6/1 -> Product6/2
  Product6/1 -> Product7/1
  Compare To Constant7/1 -> Product7/2
  Compare To Constant3/1 -> Product3/2
  Constant/1 -> Compare To Constant/1
  Compare To Constant/1 -> Product/2
  Compare To Constant1/1 -> Product1/2
  Product4/1 -> Product5/1
  Product1/1 -> Product8/2
  Product8/1 -> Bistable/1
  Product3/1 -> Product9/2
  Product5/1 -> Product10/2
  Product7/1 -> Product11/2
  Compare To Constant8/1 -> Product11/1, Product10/1, Product9/1, Product8/1
  PLL (3ph)/2 -> Compare To Constant8/1
  Voltage Measurement1/1 -> Mux1/2
  Voltage Measurement/1 -> Mux1/1
  Voltage Measurement2/1 -> Mux1/3
  Mux1/1 -> PLL (3ph)/1
  Gain/1 -> Scope1/1, Three-Phase Fault1/1
  Gain1/1 -> Scope2/1, Three-Phase Fault2/1
  Gain2/1 -> Three-Phase Fault3/1, Scope3/1
  Gain3/1 -> Scope4/1, Three-Phase Fault4/1
  Bistable/1 -> Gain/1
  Product9/1 -> Bistable1/1
  Bistable1/1 -> Gain1/1
  Bistable3/1 -> Gain2/1
  Product10/1 -> Bistable3/1
  Product11/1 -> Bistable2/1
  Bistable2/1 -> Gain3/1
  connections:
  Voltage Measurement1/LConn1 -- B/RConn1 -- Three-Phase Fault1/LConn2 -- Three-Phase Fault2/LConn2 -- Three-Phase Fault3/LConn2 -- Three-Phase Fault4/LConn2
  Voltage Measurement2/LConn1 -- C/RConn1 -- Three-Phase Fault4/LConn3 -- Three-Phase Fault3/LConn3 -- Three-Phase Fault2/LConn3 -- Three-Phase Fault1/LConn3
  A/RConn1 -- Voltage Measurement/LConn1 -- Three-Phase Fault1/LConn1 -- Three-Phase Fault2/LConn1 -- Three-Phase Fault3/LConn1 -- Three-Phase Fault4/LConn1
  Ground/LConn1 -- Voltage Measurement/LConn2
  Ground1/LConn1 -- Voltage Measurement1/LConn2
  Ground2/LConn1 -- Voltage Measurement2/LConn2

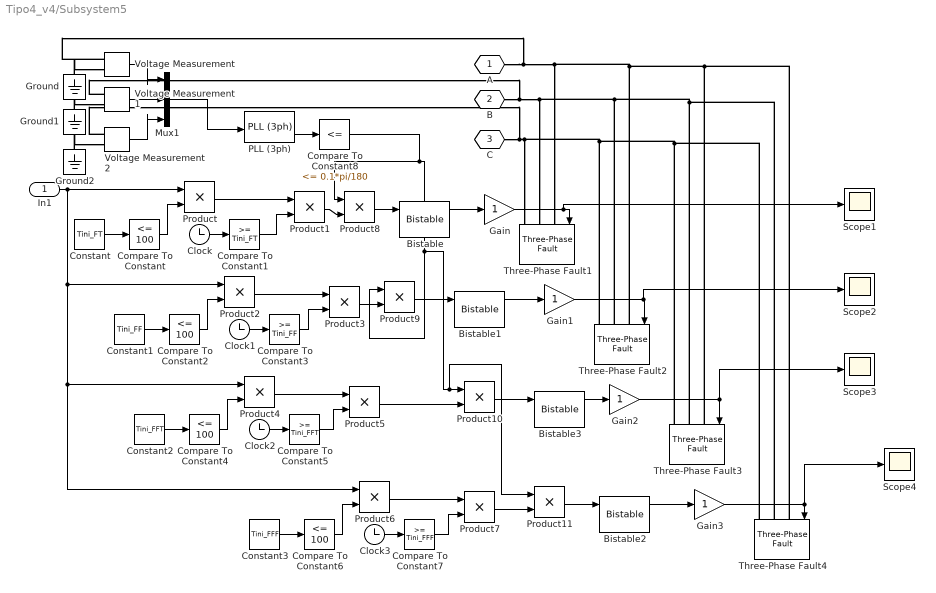
== system Tipo4_v4/Subsystem5 ==
  In1 : Inport
  Bistable{,1..3} (4 alike) : powerlib_meascontrol/Logic/Bistable  Qpriority=Set  ic=0  Ts=Ts
      settings: SourceProductName=Simscape Power Systems  SourceProductBaseCode=PS
  Clock{,1..3} (4 alike) : Clock
  Compare To Constant{,2,4,6} (4 alike) : simulink/Logic and Bit Operations/Compare To Constant  relop=<=  const=100  OutDataTypeStr=uint8
  Compare To Constant1 : simulink/Logic and Bit Operations/Compare To Constant  relop=>=  const=Tini_FT  OutDataTypeStr=uint8
  Compare To Constant3 : simulink/Logic and Bit Operations/Compare To Constant  relop=>=  const=Tini_FF  OutDataTypeStr=uint8
  Compare To Constant5 : simulink/Logic and Bit Operations/Compare To Constant  relop=>=  const=Tini_FFT  OutDataTypeStr=uint8
  Compare To Constant7 : simulink/Logic and Bit Operations/Compare To Constant  relop=>=  const=Tini_FFF  OutDataTypeStr=uint8
  Compare To Constant8 : simulink/Logic and Bit Operations/Compare To Constant  relop=<=  const=0.1*pi/180  OutDataTypeStr=uint8
  Constant : Constant  Value=Tini_FT
  Constant1 : Constant  Value=Tini_FF
  Constant2 : Constant  Value=Tini_FFT
  Constant3 : Constant  Value=Tini_FFF
  Gain{,1..3} (4 alike) : Gain  OutDataTypeStr=double
  Ground : powerlib/Elements/Ground  LConnTagsString=a
  Ground1 : powerlib/Elements/Ground  LConnTagsString=a
  Ground2 : powerlib/Elements/Ground  LConnTagsString=a
  Mux1 : Mux  Inputs=3
  PLL (3ph) : powerlib_meascontrol/PLL/PLL (3ph)  Fmin=60  Par_Init=[0, 60]  ParK=[180, 3200, 1]  TcD=1e-4  MaxRateChangeFreq=12  FilterCutOffFreq=25  Ts=Ts  AGC=on
  Product{,2..7} (7 alike) : Product
  Product{1,8..11} (5 alike) : Product  RndMeth=Ceiling
  Scope{1..4} (4 alike) : Scope
  Three-Phase Fault1 : powerlib/Elements/Three-Phase Fault  InitialStates=0  FaultA=on  FaultB=off  FaultC=off  GroundFault=on  SwitchTimes=[900 1000]  External=on  SwitchStatus=NaN  FaultResistance=R_falta  GroundResistance=R_falta  SnubberResistance=1e6  SnubberCapacitance=inf  Measurements=None
  Three-Phase Fault2 : powerlib/Elements/Three-Phase Fault  InitialStates=0  FaultA=on  FaultB=on  FaultC=off  GroundFault=off  SwitchTimes=[900 1000]  External=on  SwitchStatus=NaN  FaultResistance=R_falta  GroundResistance=1e-12  SnubberResistance=1e6  SnubberCapacitance=inf  Measurements=None
  Three-Phase Fault3 : powerlib/Elements/Three-Phase Fault  InitialStates=0  FaultA=on  FaultB=on  FaultC=off  GroundFault=on  SwitchTimes=[900 1000]  External=on  SwitchStatus=NaN  FaultResistance=R_falta  GroundResistance=R_falta  SnubberResistance=1e6  SnubberCapacitance=inf  Measurements=None
  Three-Phase Fault4 : powerlib/Elements/Three-Phase Fault  InitialStates=0  FaultA=on  FaultB=on  FaultC=on  GroundFault=on  SwitchTimes=[900 1000]  External=on  SwitchStatus=NaN  FaultResistance=R_falta  GroundResistance=R_falta  SnubberResistance=1e6  SnubberCapacitance=inf  Measurements=None
  Voltage Measurement : powerlib/Measurements/Voltage Measurement  PhasorSimulation=off  OutputType=Complex  PSBequivalent=0
  Voltage Measurement1 : powerlib/Measurements/Voltage Measurement  PhasorSimulation=off  OutputType=Complex  PSBequivalent=0
  Voltage Measurement2 : powerlib/Measurements/Voltage Measurement  PhasorSimulation=off  OutputType=Complex  PSBequivalent=0
  A : PMIOPort  Tag=PMCPort  Side=Right
  B : PMIOPort  Tag=PMCPort  Port=2  Side=Right
  C : PMIOPort  Tag=PMCPort  Port=3  Side=Right
  wires:
  Clock/1 -> Compare To Constant1/1
  Product2/1 -> Product3/1
  Constant1/1 -> Compare To Constant2/1
  Product/1 -> Product1/1
  Compare To Constant2/1 -> Product2/2
  Constant2/1 -> Compare To Constant4/1
  Clock2/1 -> Compare To Constant5/1
  Compare To Constant4/1 -> Product4/2
  Clock1/1 -> Compare To Constant3/1
  Compare To Constant5/1 -> Product5/2
  In1/1 -> Product/1, Product2/1, Product4/1, Product6/1
  Clock3/1 -> Compare To Constant7/1
  Constant3/1 -> Compare To Constant6/1
  Compare To Constant6/1 -> Product6/2
  Product6/1 -> Product7/1
  Compare To Constant7/1 -> Product7/2
  Compare To Constant3/1 -> Product3/2
  Constant/1 -> Compare To Constant/1
  Compare To Constant/1 -> Product/2
  Compare To Constant1/1 -> Product1/2
  Product4/1 -> Product5/1
  Product1/1 -> Product8/2
  Product8/1 -> Bistable/1
  Product3/1 -> Product9/2
  Product5/1 -> Product10/2
  Product7/1 -> Product11/2
  Compare To Constant8/1 -> Product11/1, Product10/1, Product9/1, Product8/1
  PLL (3ph)/2 -> Compare To Constant8/1
  Voltage Measurement1/1 -> Mux1/2
  Voltage Measurement/1 -> Mux1/1
  Voltage Measurement2/1 -> Mux1/3
  Mux1/1 -> PLL (3ph)/1
  Gain/1 -> Scope1/1, Three-Phase Fault1/1
  Gain1/1 -> Scope2/1, Three-Phase Fault2/1
  Gain2/1 -> Three-Phase Fault3/1, Scope3/1
  Gain3/1 -> Scope4/1, Three-Phase Fault4/1
  Bistable/1 -> Gain/1
  Product9/1 -> Bistable1/1
  Bistable1/1 -> Gain1/1
  Bistable3/1 -> Gain2/1
  Product10/1 -> Bistable3/1
  Product11/1 -> Bistable2/1
  Bistable2/1 -> Gain3/1
  connections:
  Voltage Measurement1/LConn1 -- B/RConn1 -- Three-Phase Fault1/LConn2 -- Three-Phase Fault2/LConn2 -- Three-Phase Fault3/LConn2 -- Three-Phase Fault4/LConn2
  Voltage Measurement2/LConn1 -- C/RConn1 -- Three-Phase Fault4/LConn3 -- Three-Phase Fault3/LConn3 -- Three-Phase Fault2/LConn3 -- Three-Phase Fault1/LConn3
  A/RConn1 -- Voltage Measurement/LConn1 -- Three-Phase Fault1/LConn1 -- Three-Phase Fault2/LConn1 -- Three-Phase Fault3/LConn1 -- Three-Phase Fault4/LConn1
  Ground/LConn1 -- Voltage Measurement/LConn2
  Ground1/LConn1 -- Voltage Measurement1/LConn2
  Ground2/LConn1 -- Voltage Measurement2/LConn2

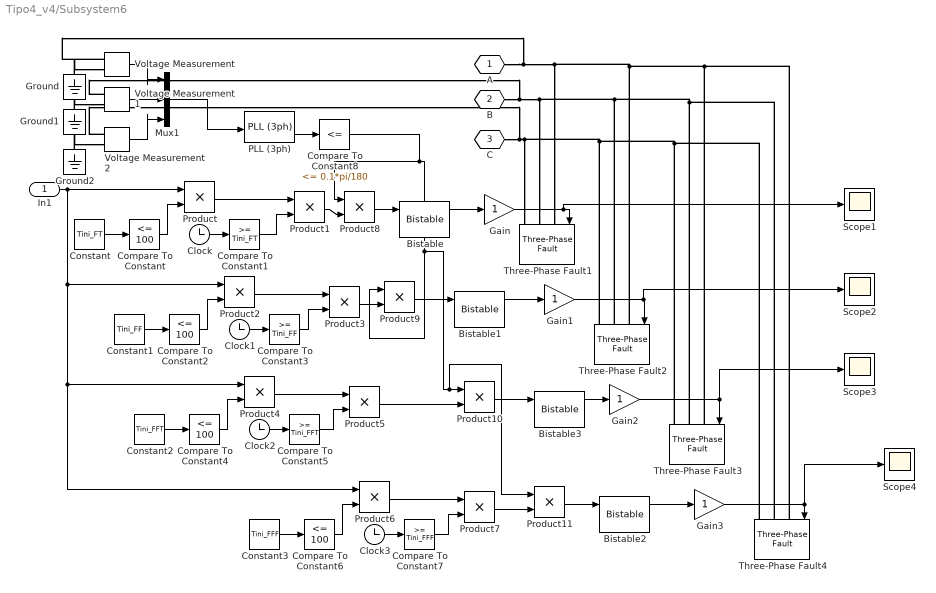
== system Tipo4_v4/Subsystem6 ==
  In1 : Inport
  Bistable{,1..3} (4 alike) : powerlib_meascontrol/Logic/Bistable  Qpriority=Set  ic=0  Ts=Ts
      settings: SourceProductName=Simscape Power Systems  SourceProductBaseCode=PS
  Clock{,1..3} (4 alike) : Clock
  Compare To Constant{,2,4,6} (4 alike) : simulink/Logic and Bit Operations/Compare To Constant  relop=<=  const=100  OutDataTypeStr=uint8
  Compare To Constant1 : simulink/Logic and Bit Operations/Compare To Constant  relop=>=  const=Tini_FT  OutDataTypeStr=uint8
  Compare To Constant3 : simulink/Logic and Bit Operations/Compare To Constant  relop=>=  const=Tini_FF  OutDataTypeStr=uint8
  Compare To Constant5 : simulink/Logic and Bit Operations/Compare To Constant  relop=>=  const=Tini_FFT  OutDataTypeStr=uint8
  Compare To Constant7 : simulink/Logic and Bit Operations/Compare To Constant  relop=>=  const=Tini_FFF  OutDataTypeStr=uint8
  Compare To Constant8 : simulink/Logic and Bit Operations/Compare To Constant  relop=<=  const=0.1*pi/180  OutDataTypeStr=uint8
  Constant : Constant  Value=Tini_FT
  Constant1 : Constant  Value=Tini_FF
  Constant2 : Constant  Value=Tini_FFT
  Constant3 : Constant  Value=Tini_FFF
  Gain{,1..3} (4 alike) : Gain  OutDataTypeStr=double
  Ground : powerlib/Elements/Ground  LConnTagsString=a
  Ground1 : powerlib/Elements/Ground  LConnTagsString=a
  Ground2 : powerlib/Elements/Ground  LConnTagsString=a
  Mux1 : Mux  Inputs=3
  PLL (3ph) : powerlib_meascontrol/PLL/PLL (3ph)  Fmin=60  Par_Init=[0, 60]  ParK=[180, 3200, 1]  TcD=1e-4  MaxRateChangeFreq=12  FilterCutOffFreq=25  Ts=Ts  AGC=on
  Product{,2..7} (7 alike) : Product
  Product{1,8..11} (5 alike) : Product  RndMeth=Ceiling
  Scope{1..4} (4 alike) : Scope
  Three-Phase Fault1 : powerlib/Elements/Three-Phase Fault  InitialStates=0  FaultA=on  FaultB=off  FaultC=off  GroundFault=on  SwitchTimes=[900 1000]  External=on  SwitchStatus=NaN  FaultResistance=R_falta  GroundResistance=R_falta  SnubberResistance=1e6  SnubberCapacitance=inf  Measurements=None
  Three-Phase Fault2 : powerlib/Elements/Three-Phase Fault  InitialStates=0  FaultA=on  FaultB=on  FaultC=off  GroundFault=off  SwitchTimes=[900 1000]  External=on  SwitchStatus=NaN  FaultResistance=R_falta  GroundResistance=1e-12  SnubberResistance=1e6  SnubberCapacitance=inf  Measurements=None
  Three-Phase Fault3 : powerlib/Elements/Three-Phase Fault  InitialStates=0  FaultA=on  FaultB=on  FaultC=off  GroundFault=on  SwitchTimes=[900 1000]  External=on  SwitchStatus=NaN  FaultResistance=R_falta  GroundResistance=R_falta  SnubberResistance=1e6  SnubberCapacitance=inf  Measurements=None
  Three-Phase Fault4 : powerlib/Elements/Three-Phase Fault  InitialStates=0  FaultA=on  FaultB=on  FaultC=on  GroundFault=on  SwitchTimes=[900 1000]  External=on  SwitchStatus=NaN  FaultResistance=R_falta  GroundResistance=R_falta  SnubberResistance=1e6  SnubberCapacitance=inf  Measurements=None
  Voltage Measurement : powerlib/Measurements/Voltage Measurement  PhasorSimulation=off  OutputType=Complex  PSBequivalent=0
  Voltage Measurement1 : powerlib/Measurements/Voltage Measurement  PhasorSimulation=off  OutputType=Complex  PSBequivalent=0
  Voltage Measurement2 : powerlib/Measurements/Voltage Measurement  PhasorSimulation=off  OutputType=Complex  PSBequivalent=0
  A : PMIOPort  Tag=PMCPort  Side=Right
  B : PMIOPort  Tag=PMCPort  Port=2  Side=Right
  C : PMIOPort  Tag=PMCPort  Port=3  Side=Right
  wires:
  Clock/1 -> Compare To Constant1/1
  Product2/1 -> Product3/1
  Constant1/1 -> Compare To Constant2/1
  Product/1 -> Product1/1
  Compare To Constant2/1 -> Product2/2
  Constant2/1 -> Compare To Constant4/1
  Clock2/1 -> Compare To Constant5/1
  Compare To Constant4/1 -> Product4/2
  Clock1/1 -> Compare To Constant3/1
  Compare To Constant5/1 -> Product5/2
  In1/1 -> Product/1, Product2/1, Product4/1, Product6/1
  Clock3/1 -> Compare To Constant7/1
  Constant3/1 -> Compare To Constant6/1
  Compare To Constant6/1 -> Product6/2
  Product6/1 -> Product7/1
  Compare To Constant7/1 -> Product7/2
  Compare To Constant3/1 -> Product3/2
  Constant/1 -> Compare To Constant/1
  Compare To Constant/1 -> Product/2
  Compare To Constant1/1 -> Product1/2
  Product4/1 -> Product5/1
  Product1/1 -> Product8/2
  Product8/1 -> Bistable/1
  Product3/1 -> Product9/2
  Product5/1 -> Product10/2
  Product7/1 -> Product11/2
  Compare To Constant8/1 -> Product11/1, Product10/1, Product9/1, Product8/1
  PLL (3ph)/2 -> Compare To Constant8/1
  Voltage Measurement1/1 -> Mux1/2
  Voltage Measurement/1 -> Mux1/1
  Voltage Measurement2/1 -> Mux1/3
  Mux1/1 -> PLL (3ph)/1
  Gain/1 -> Scope1/1, Three-Phase Fault1/1
  Gain1/1 -> Scope2/1, Three-Phase Fault2/1
  Gain2/1 -> Three-Phase Fault3/1, Scope3/1
  Gain3/1 -> Scope4/1, Three-Phase Fault4/1
  Bistable/1 -> Gain/1
  Product9/1 -> Bistable1/1
  Bistable1/1 -> Gain1/1
  Bistable3/1 -> Gain2/1
  Product10/1 -> Bistable3/1
  Product11/1 -> Bistable2/1
  Bistable2/1 -> Gain3/1
  connections:
  Voltage Measurement1/LConn1 -- B/RConn1 -- Three-Phase Fault1/LConn2 -- Three-Phase Fault2/LConn2 -- Three-Phase Fault3/LConn2 -- Three-Phase Fault4/LConn2
  Voltage Measurement2/LConn1 -- C/RConn1 -- Three-Phase Fault4/LConn3 -- Three-Phase Fault3/LConn3 -- Three-Phase Fault2/LConn3 -- Three-Phase Fault1/LConn3
  A/RConn1 -- Voltage Measurement/LConn1 -- Three-Phase Fault1/LConn1 -- Three-Phase Fault2/LConn1 -- Three-Phase Fault3/LConn1 -- Three-Phase Fault4/LConn1
  Ground/LConn1 -- Voltage Measurement/LConn2
  Ground1/LConn1 -- Voltage Measurement1/LConn2
  Ground2/LConn1 -- Voltage Measurement2/LConn2
